simulink model "arduino_pid_2018a"  (R2018a)
settings: Solver=ode3  StartTime=0.0  StopTime=10  FixedStep=0.01  RelTol=1e-3  EnableMultiTasking=on
undefined symbols (not defined in the file): DiscIntNeverNeededParam
libraries: pil_lib x2, simulink x1
settings Model: SimulationMode=processor-in-the-loop (pil)  ExtModeTrigDuration=2  Creator=jedsada-emertxe  LastModifiedBy=jedsada-emertxe
settings SolverCC: PositivePriorityOrder=on
settings DataIOCC: SaveFormat=Array  ReturnWorkspaceOutputs=on
settings OptimizationCC: UseDivisionForNetSlopeComputation=UseDivisionForReciprocalsOfIntegersOnly  EnhancedBackFolding=on  PassReuseOutputArgsAs=Individual arguments  ZeroExternalMemoryAtStartup=off  ZeroInternalMemoryAtStartup=off  MaxStackSize=64  OptimizeBlockOrder=speed  DifferentSizesBufferReuse=on  OptimizationCustomize=off
settings DebuggingCC: ParameterTunabilityLossMsg=error
settings HardwareCC: ProdBitPerInt=16  ProdBitPerPointer=16  ProdBitPerSizeT=16  ProdBitPerPtrDiffT=16  ProdLargestAtomicFloat=None  ProdWordSize=8  ProdHWDeviceType=Atmel->AVR  TargetBitPerPointer=64  TargetBitPerSizeT=64  TargetBitPerPtrDiffT=64  TargetLongLongMode=on  TargetIntDivRoundTo=Zero  TargetEndianess=LittleEndian  TargetWordSize=64  TargetHWDeviceType=MATLAB Host  ProdEqTarget=off
settings ModelReferenceCC: PropagateSignalLabelsOutOfModel=off
settings SFSimCC: MATLABDynamicMemAlloc=off
settings RTWCC: SystemTargetFile=ert.tlc  HardwareBoard=Arduino Uno  TLCOptions=-aInlineSetEventsForThisBaseRateFcn=TLC_FALSE -aSuppressMultiTaskScheduler=TLC_FALSE -aRateBasedStepFcn=1  TemplateMakefile=ert_default_tmf  GenerateReport=on  Toolchain=Arduino AVR  BuildConfiguration=Faster Runs  IncludeHyperlinkInReport=on  LaunchReport=on  GenerateTraceInfo=on  GenerateTraceReport=on  GenerateTraceReportSl=on  GenerateTraceReportSf=on  GenerateTraceReportEml=on  GenerateCodeMetricsReport=on
settings CodeAppCC: ForceParamTrailComments=on  IgnoreCustomStorageClasses=off  IgnoreTestpoints=on  OperatorAnnotations=on  SimulinkDataObjDesc=on  SFDataObjDesc=on  InsertBlockDesc=on
settings ERTTargetCC: SupportContinuousTime=on  SupportVariableSizeSignals=on

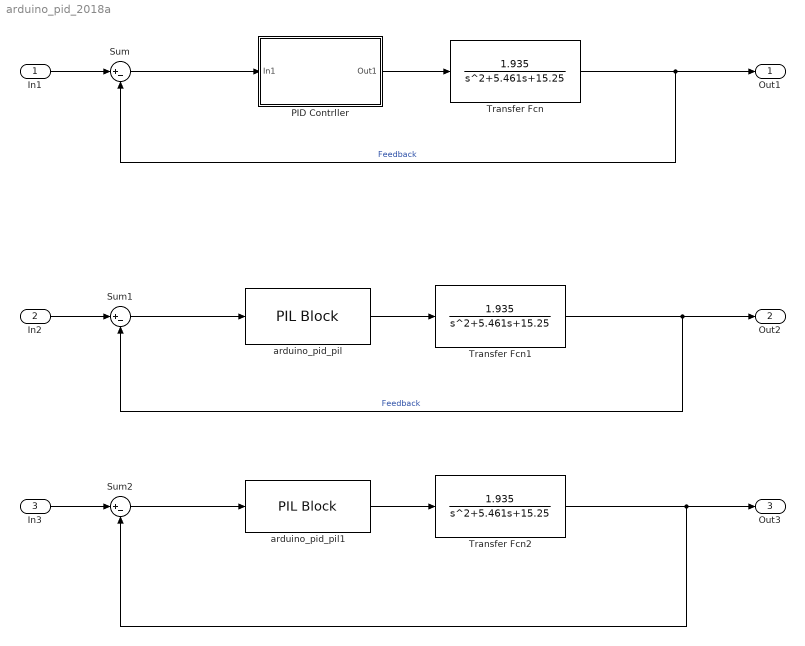
== system arduino_pid_2018a ==
  In1 : Inport
  In2 : Inport  Port=2
  In3 : Inport  Port=3
  PID Contrller : Subsystem
  Sum : Sum  Inputs=|+-
  Sum1 : Sum  Inputs=|+-
  Sum2 : Sum  Inputs=|+-
  Transfer Fcn : TransferFcn  Numerator=[1.935]  Denominator=[1 5.461 15.25]
  Transfer Fcn1 : TransferFcn  Numerator=[1.935]  Denominator=[1 5.461 15.25]
  Transfer Fcn2 : TransferFcn  Numerator=[1.935]  Denominator=[1 5.461 15.25]
  arduino_pid_pil : pil_lib/PIL Block  SimulationMode=SIL  IsTopModelPIL=on  CodeDir=C:\WorkSpace\arduino_pid_pil_ert_rtw  AnchorDir=C:\WorkSpace  ConfigName=Software-in-the-Loop (SIL)  XrelIsTopModelCode=on  XrelIsReusable=off  XrelDWorkNames={}  XrelDWorkTypes={}  XrelModelArgVals={}  XrelOrderedParamNames={}
  arduino_pid_pil1 : pil_lib/PIL Block  SimulationMode=PIL  IsTopModelPIL=on  CodeDir=C:\WorkSpace\arduino_pid_pil_ert_rtw  AnchorDir=C:\WorkSpace  ConfigName=Arduino Board  XrelIsTopModelCode=on  XrelIsReusable=off  XrelDWorkNames={}  XrelDWorkTypes={}  XrelModelArgVals={}  XrelOrderedParamNames={}
  Out1 : Outport
  Out2 : Outport  Port=2
  Out3 : Outport  Port=3
  wires:
  PID Contrller/1(Out1) -> Transfer Fcn/1
  Transfer Fcn/1 -> Sum/2, Out1/1  "Feedback"
  arduino_pid_pil/1 -> Transfer Fcn1/1
  Transfer Fcn1/1 -> Sum1/2, Out2/1  "Feedback"
  In1/1 -> Sum/1
  Sum/1 -> PID Contrller/1(In1)
  In2/1 -> Sum1/1
  Sum1/1 -> arduino_pid_pil/1
  In3/1 -> Sum2/1
  Sum2/1 -> arduino_pid_pil1/1
  arduino_pid_pil1/1 -> Transfer Fcn2/1
  Transfer Fcn2/1 -> Sum2/2, Out3/1

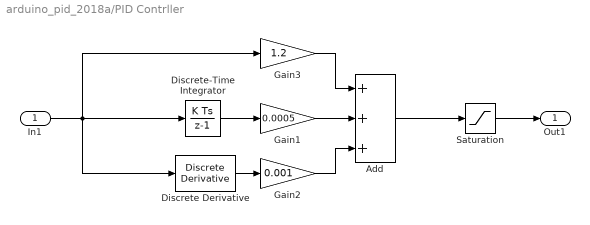
== system arduino_pid_2018a/PID Contrller ==
  In1 : Inport
  Add : Sum  Inputs=+++
  Discrete Derivative : simulink/Discrete/Discrete Derivative  gainval=1.0  ICPrevScaledInput=0.0  OutMin=[]  OutMax=[]  OutDataType=fixdt(1, 16)  OutScaling=2^-10  DoSatur=off
  Discrete-Time Integrator : DiscreteIntegrator  SampleTime=-1  ICPrevOutput=DiscIntNeverNeededParam  ICPrevScaledInput=DiscIntNeverNeededParam
  Gain1 : Gain  Gain=0.0005
  Gain2 : Gain  Gain=0.001
  Gain3 : Gain  Gain=1.2
  Saturation : Saturate  UpperLimit=255  LowerLimit=0
  Out1 : Outport
  wires:
  Discrete Derivative/1 -> Gain2/1
  In1/1 -> Gain3/1, Discrete Derivative/1, Discrete-Time Integrator/1
  Gain2/1 -> Add/3
  Gain3/1 -> Add/1
  Discrete-Time Integrator/1 -> Gain1/1
  Add/1 -> Saturation/1
  Gain1/1 -> Add/2
  Saturation/1 -> Out1/1
